simulink model "q3w8"  (R2014b)
settings: Solver=ode23  StartTime=0.0  StopTime=1.0  RelTol=1e-3
values from neighbouring files (symbols this model uses):
  Bm = 0.83e-3    (= 0.00083)    [ardat1.m]    (also in ardat2.m)
  Ea = 230    [ardat1.m]    (also in ardat2.m = 200)
  Jm = 0.068    [ardat1.m]    (also in ardat2.m = 0.00286)
  Kb = Ki    (= 1.0712)    [ardat1.m]    (also in ardat2.m = 1.42857)
  Ki = 1.0712    [ardat1.m]    (also in ardat2.m = 1.42857)
  La = 4.5e-3    (= 0.0045)    [ardat1.m]    (also in ardat2.m = 0.4549)
  Ra = .615    (= 0.615)    [ardat1.m]    (also in ardat2.m = 16.105)
  Tl = 20    [ardat1.m]    (also in ardat2.m = 2)
settings Model: Creator=Student  LastModifiedBy=Student

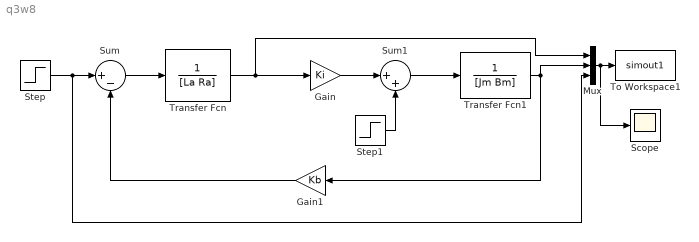
== system q3w8 ==
  Gain : Gain  Gain=Ki
  Gain1 : Gain  Gain=Kb
  Mux : Mux  Inputs=3
  Scope : Scope
      settings: ShowLegends=on
  Step : Step  Time=0.2  After=Ea  SampleTime=0
  Step1 : Step  Time=0.2  After=Tl  SampleTime=0
  Sum : Sum  Inputs=|+-
  Sum1 : Sum  Inputs=|++
  To Workspace1 : ToWorkspace  VariableName=simout1  SaveFormat=Timeseries  SampleTime=-1
  Transfer Fcn : TransferFcn  Denominator=[La Ra]
  Transfer Fcn1 : TransferFcn  Denominator=[Jm Bm]
  wires:
  Transfer Fcn/1 -> Mux/1, Gain/1
  Gain/1 -> Sum1/1
  Sum1/1 -> Transfer Fcn1/1
  Transfer Fcn1/1 -> Gain1/1, Mux/2
  Gain1/1 -> Sum/2
  Sum/1 -> Transfer Fcn/1
  Step1/1 -> Sum1/2
  Step/1 -> Mux/3, Sum/1
  Mux/1 -> Scope/1, To Workspace1/1
